simulink model "VTOL_animation"  (R2015a)
settings: Solver=ode45  StartTime=0.0  StopTime=10000  RelTol=1e-3
undefined symbols (not defined in the file or in its folder): drawVTOL
libraries: simulink x4
settings Model: Creator=beard  LastModifiedBy=beard
settings DataIOCC: SignalLoggingSaveFormat=ModelDataLogs
settings OptimizationCC: ExpressionDepthLimit=2147483647  InitFltsAndDblsToZero=on
settings DebuggingCC: UnderspecifiedInitializationDetection=Classic  MergeDetectMultiDrivingBlocksExec=none  SolverPrmCheckMsg=warning  FcnCallInpInsideContextMsg=UseLocalSettings  StateNameClashWarn=warning
settings GRTTargetCC: CombineOutputUpdateFcns=off  GRTInterface=on

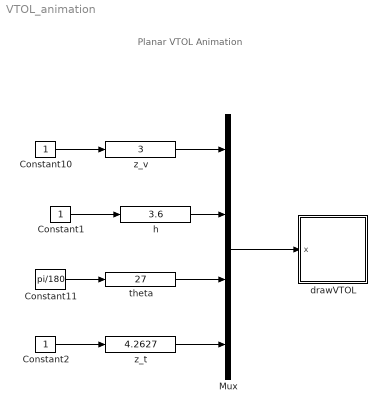
== system VTOL_animation ==
  note: Planar VTOL Animation
  Constant1 : Constant
  Constant10 : Constant
  Constant11 : Constant  Value=pi/180
  Constant2 : Constant
  Mux : Mux
  drawVTOL : Subsystem
      mask Display: image(imread('tv.jpg'))
  h : simulink/Math Operations/Slider Gain  low=0  gain=3.6  high=10
  theta : simulink/Math Operations/Slider Gain  low=-90  gain=27  high=90
  z_t : simulink/Math Operations/Slider Gain  low=0  gain=4.2627  high=5
  z_v : simulink/Math Operations/Slider Gain  low=0  gain=3  high=10
  wires:
  z_v/1 -> Mux/1
  Constant10/1 -> z_v/1
  theta/1 -> Mux/3
  Constant11/1 -> theta/1
  Mux/1 -> drawVTOL/1(x)
  Constant1/1 -> h/1
  h/1 -> Mux/2
  Constant2/1 -> z_t/1
  z_t/1 -> Mux/4

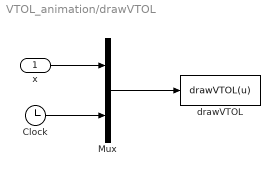
== system VTOL_animation/drawVTOL ==
  x : Inport
  Clock : Clock
  Mux : Mux  Inputs=2
  drawVTOL : MATLABFcn  MATLABFcn=drawVTOL(u)  OutputDimensions=0  SampleTime=0.1
  wires:
  Mux/1 -> drawVTOL/1
  x/1 -> Mux/1
  Clock/1 -> Mux/2
